simulink model "base_1fm"  (R2016b)
settings: Solver=VariableStepAuto  StartTime=0.0  StopTime=10.0  RelTol=1e-3
values from neighbouring files (symbols this model uses):
  Lb = 0.07    [base_1fm_parameters.m]
  Lf = 0.238    [base_1fm_parameters.m]
  Lu = 0.153    [base_1fm_parameters.m]
  sampleTime = 0.001    [base_1fm_parameters.m]
undefined symbols (not defined in the file or in its folder): DiscIntNeverNeededParam, RobotStruct
undefined symbols (not defined in the file): RobotStruct_FM1
libraries: simulink x27, VariousBlocksLibrary x4, FMLibrary_v2 x2, UsefulBlocksLibrary x2, simulink_extras x2, FM_Library x1
(part 1 of 3)
settings Model: Creator=niekbeckers  LastModifiedBy=niekbeckers

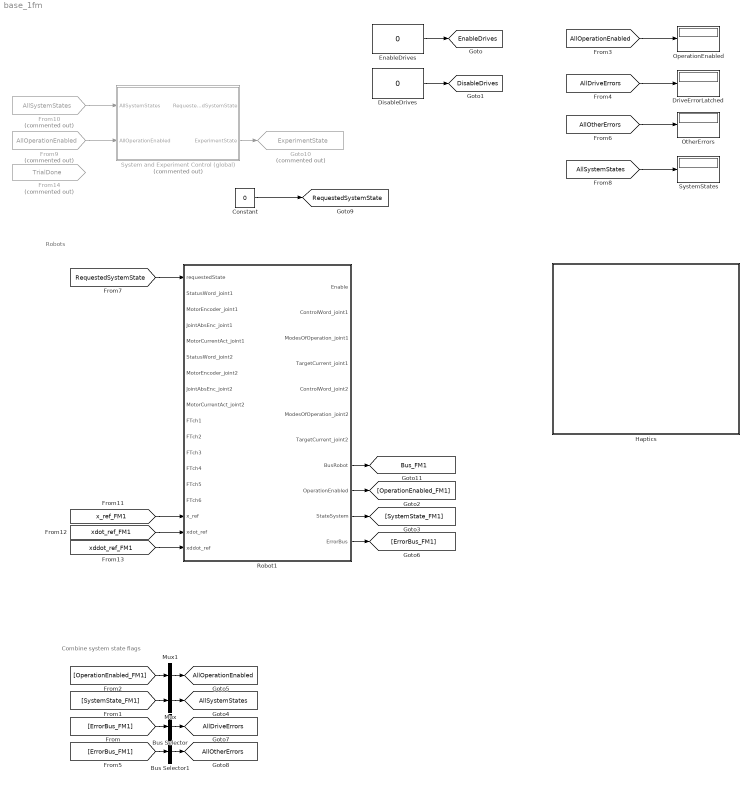
== system base_1fm ==
  note: Combine system state flags
  note: Robots
  Bus Selector : BusSelector  OutputSignals=DriveErrorLatched  OutputAsBus=on
  Bus Selector1 : BusSelector  OutputSignals=WorkspaceErrorLatched,ForceSensorLatched  OutputAsBus=on
  Constant : Constant  Value=0
  DisableDrives : Constant  Value=0
      settings: OpenFcn=set_param(gcb,'Value','1');tname = ['toggletimer_' gcb];delete(timerfind('name',tname));t = timer('timerfcn', ['set_param(''',gcb,''',''Value'',''0'')'],'executionmode','singleshot','startdelay',1,'name',tname);start(t);
      mask Display: fprintf('PushToTrigger\n%s',get_param(gcb,'value'))
  DriveErrorLatched : Display
  EnableDrives : Constant  Value=0
      settings: OpenFcn=set_param(gcb,'Value','1');tname = ['toggletimer_' gcb];delete(timerfind('name',tname));t = timer('timerfcn', ['set_param(''',gcb,''',''Value'',''0'')'],'executionmode','singleshot','startdelay',1,'name',tname);start(t);
      mask Display: fprintf('PushToTrigger\n%s',get_param(gcb,'value'))
  From10 : From  Commented=on  GotoTag=AllSystemStates
  From14 : From  Commented=on  GotoTag=TrialDone
  From9 : From  Commented=on  GotoTag=AllOperationEnabled
  Goto10 : Goto  Commented=on  GotoTag=ExperimentState  TagVisibility=global
  Haptics : Subsystem
  Mux : Mux  Inputs=1
  Mux1 : Mux  Inputs=1
  OperationEnabled : Display
  OtherErrors : Display
  Robot1 : Subsystem  mask{RobotStruct=RobotStruct_FM1}
      mask prompts: RobotStruct "Robot struct (data)"
  System and Experiment Control (global) : Subsystem  Commented=on
  SystemStates : Display
  tag scope: AllDriveErrors=global, AllOperationEnabled=global, AllOtherErrors=global, AllSystemStates=global, Bus_FM1=global, DisableDrives=global, EnableDrives=global, RequestedSystemState=global
  wires:
  DisableDrives/1 -> [DisableDrives]
  EnableDrives/1 -> [EnableDrives]
  Robot1/9(OperationEnabled) -> [OperationEnabled_FM1]
  [AllOperationEnabled] -> OperationEnabled/1
  Robot1/10(StateSystem) -> [SystemState_FM1]
  [SystemState_FM1] -> Mux/1
  Mux/1 -> [AllSystemStates]
  Mux1/1 -> [AllOperationEnabled]
  [OperationEnabled_FM1] -> Mux1/1
  Robot1/11(ErrorBus) -> [ErrorBus_FM1]
  [ErrorBus_FM1] -> Bus Selector/1
  Bus Selector/1 -> [AllDriveErrors]
  [AllDriveErrors] -> DriveErrorLatched/1
  [ErrorBus_FM1] -> Bus Selector1/1
  Bus Selector1/1 -> [AllOtherErrors]
  [AllOtherErrors] -> OtherErrors/1
  [RequestedSystemState] -> Robot1/1(requestedState)
  [AllSystemStates] -> SystemStates/1
  System and Experiment Control (global)/2(ExperimentState) -> Goto10/1
  From10/1 -> System and Experiment Control (global)/1(AllSystemStates)
  From9/1 -> System and Experiment Control (global)/2(AllOperationEnabled)
  [x_ref_FM1] -> Robot1/16(x_ref)
  [xdot_ref_FM1] -> Robot1/17(xdot_ref)
  [xddot_ref_FM1] -> Robot1/18(xddot_ref)
  Constant/1 -> [RequestedSystemState]
  Robot1/8(BusRobot) -> [Bus_FM1]

== system base_1fm/Haptics ==
  note: Only run trajectory if all systems are in state 4 (run)
  Add : Sum
  "Check state " : simulink/Logic and Bit Operations/Compare To Constant  relop===  const=4  OutDataTypeStr=boolean
  Constant : Constant  Value=RobotStruct.HomeLocationOpSpace
  From9 : From  Commented=on  GotoTag=ExperimentState
  Goto1 : Goto  Commented=on  GotoTag=TrialDone  TagVisibility=global
  Hypotrochoid trajectory for AFFC : Subsystem
  Logical Operator : Logic  Inputs=1  AllPortsSameDT=off  OutDataTypeStr=boolean
  Terminator : Terminator
  Terminator1 : Terminator  Commented=on
  tag scope: x_ref_FM1=global, xddot_ref_FM1=global, xdot_ref_FM1=global
  wires:
  [Bus_FM1] -> Terminator/1
  Constant/1 -> Add/1
  Hypotrochoid trajectory for AFFC/1(dx_ref) -> Add/2
  Add/1 -> [x_ref_FM1]
  Hypotrochoid trajectory for AFFC/2(dxdot_ref) -> [xdot_ref_FM1]
  Hypotrochoid trajectory for AFFC/3(dxddot_ref) -> [xddot_ref_FM1]
  [AllSystemStates] -> "Check state "/1
  "Check state "/1 -> Logical Operator/1
  Logical Operator/1 -> Hypotrochoid trajectory for AFFC/Enable
  From9/1 -> Terminator1/1

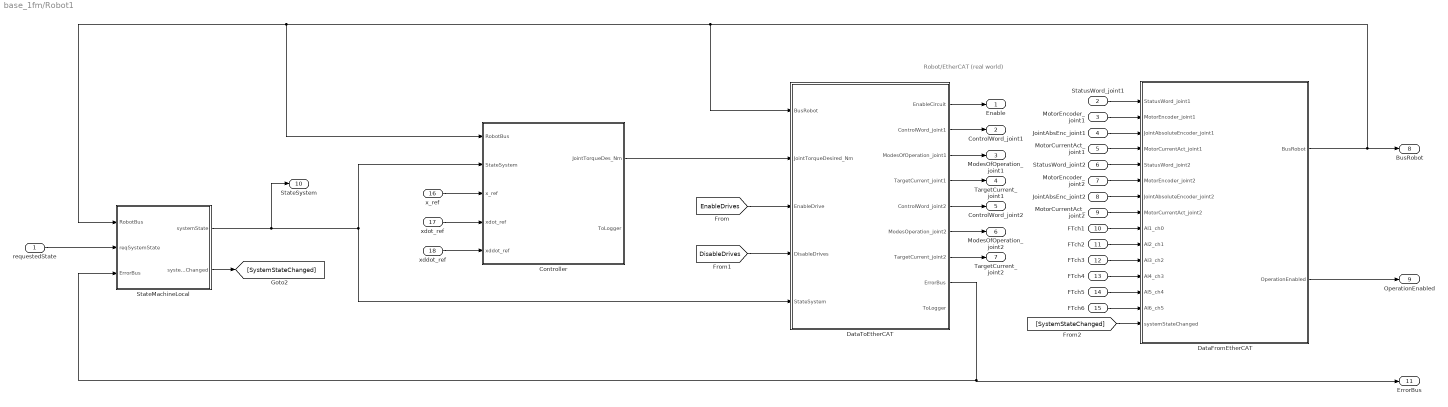
== system base_1fm/Robot1 ==
  note: Robot/EtherCAT (real world)
  requestedState : Inport
  StatusWord_joint1 : Inport  Port=2
  MotorEncoder_joint1 : Inport  Port=3
  JointAbsEnc_joint1 : Inport  Port=4
  MotorCurrentAct_joint1 : Inport  Port=5
  StatusWord_joint2 : Inport  Port=6
  MotorEncoder_joint2 : Inport  Port=7
  JointAbsEnc_joint2 : Inport  Port=8
  MotorCurrentAct_joint2 : Inport  Port=9
  FTch1 : Inport  Port=10
  FTch2 : Inport  Port=11
  FTch3 : Inport  Port=12
  FTch4 : Inport  Port=13
  FTch5 : Inport  Port=14
  FTch6 : Inport  Port=15
  x_ref : Inport  Port=16
  xdot_ref : Inport  Port=17
  xddot_ref : Inport  Port=18
  Controller : Subsystem  AncestorBlock=FMLibrary_v2/Controller
  DataFromEtherCAT : Subsystem  AncestorBlock=FMLibrary_v2/DataFromEtherCAT_FM
  DataToEtherCAT : Subsystem  AncestorBlock=FMLibrary_v2/DataToEtherCAT_FM
  StateMachineLocal : Subsystem  AncestorBlock=FMLibrary_v2/StateMachineLocal
  Enable : Outport
  ControlWord_joint1 : Outport  Port=2
  ModesOfOperation_joint1 : Outport  Port=3
  TargetCurrent_joint1 : Outport  Port=4
  ControlWord_joint2 : Outport  Port=5
  ModesOfOperation_joint2 : Outport  Port=6
  TargetCurrent_joint2 : Outport  Port=7
  BusRobot : Outport  Port=8
  OperationEnabled : Outport  Port=9
  StateSystem : Outport  Port=10
  ErrorBus : Outport  Port=11
  wires:
  DataFromEtherCAT/2(OperationEnabled) -> OperationEnabled/1
  FTch3/1 -> DataFromEtherCAT/11(AI3_ch2)
  FTch4/1 -> DataFromEtherCAT/12(AI4_ch3)
  FTch6/1 -> DataFromEtherCAT/14(AI6_ch5)
  StatusWord_joint2/1 -> DataFromEtherCAT/5(StatusWord_joint2)
  StatusWord_joint1/1 -> DataFromEtherCAT/1(StatusWord_joint1)
  DataToEtherCAT/6(ModesOperation_joint2) -> ModesOfOperation_joint2/1
  DataToEtherCAT/5(ControlWord_joint2) -> ControlWord_joint2/1
  MotorEncoder_joint1/1 -> DataFromEtherCAT/2(MotorEncoder_joint1)
  JointAbsEnc_joint2/1 -> DataFromEtherCAT/7("JointAbsoluteEncoder_joint2 ")
  FTch5/1 -> DataFromEtherCAT/13(AI5_ch4)
  DataToEtherCAT/4(TargetCurrent_joint1) -> TargetCurrent_joint1/1
  MotorCurrentAct_joint2/1 -> DataFromEtherCAT/8(MotorCurrentAct_joint2)
  [EnableDrives] -> DataToEtherCAT/3(EnableDrive)
  [DisableDrives] -> DataToEtherCAT/4(DisableDrives)
  Controller/1(JointTorqueDes_Nm) -> DataToEtherCAT/2(JointTorqueDesired_Nm)
  requestedState/1 -> StateMachineLocal/2(reqSystemState)
  DataFromEtherCAT/1(BusRobot) -> BusRobot/1, DataToEtherCAT/1(BusRobot), Controller/1(RobotBus), StateMachineLocal/1(RobotBus)
  DataToEtherCAT/8(ErrorBus) -> ErrorBus/1, StateMachineLocal/3(ErrorBus)
  [SystemStateChanged] -> DataFromEtherCAT/15(systemStateChanged)
  StateMachineLocal/2(systemStateChanged) -> [SystemStateChanged]
  DataToEtherCAT/2(ControlWord_joint1) -> ControlWord_joint1/1
  StateMachineLocal/1(systemState) -> StateSystem/1, DataToEtherCAT/5(StateSystem), Controller/2(StateSystem)
  FTch1/1 -> DataFromEtherCAT/9(AI1_ch0)
  DataToEtherCAT/1(EnableCircuit) -> Enable/1
  DataToEtherCAT/3(ModesOfOperation_joint1) -> ModesOfOperation_joint1/1
  JointAbsEnc_joint1/1 -> DataFromEtherCAT/3(JointAbsoluteEncoder_joint1)
  MotorEncoder_joint2/1 -> DataFromEtherCAT/6(MotorEncoder_joint2)
  MotorCurrentAct_joint1/1 -> DataFromEtherCAT/4(MotorCurrentAct_joint1)
  FTch2/1 -> DataFromEtherCAT/10(AI2_ch1)
  DataToEtherCAT/7(TargetCurrent_joint2) -> TargetCurrent_joint2/1
  x_ref/1 -> Controller/3(x_ref)
  xdot_ref/1 -> Controller/4(xdot_ref)
  xddot_ref/1 -> Controller/5(xddot_ref)

== system base_1fm/System and Experiment Control (global) ==
  note: Hier ergens experiment protocol inlezen
  AllSystemStates : Inport
  AllOperationEnabled : Inport  Port=2
  GlobalStateMachine : FMLibrary_v2/StateMachineLocal/SystemLocalStateMachine
  RequestedSystemState : Outport
  ExperimentState : Outport  Port=2
  wires:
  GlobalStateMachine/1 -> RequestedSystemState/1

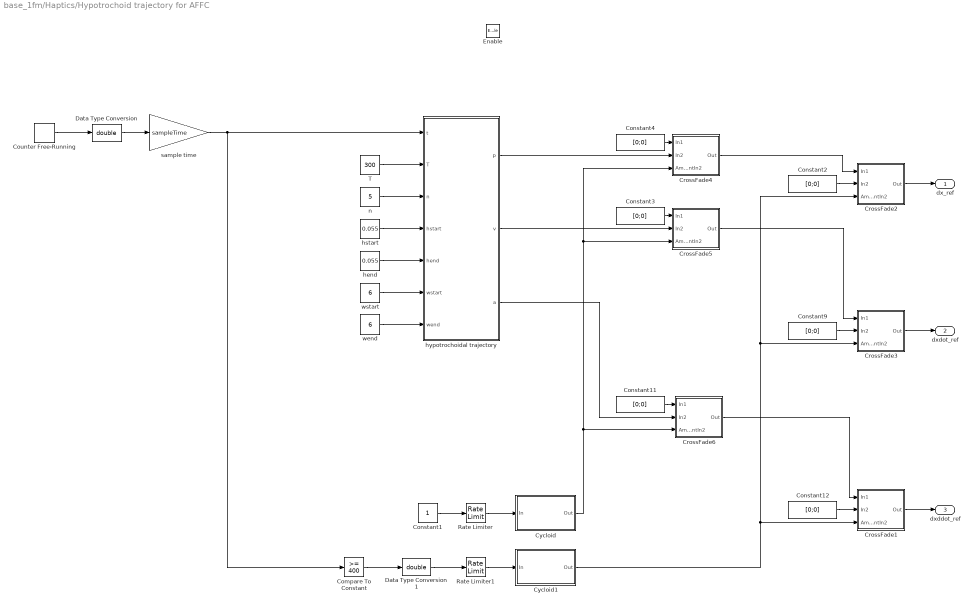
== system base_1fm/Haptics/Hypotrochoid trajectory for AFFC ==
  Enable : EnablePort  StatesWhenEnabling=reset
  Compare To Constant : simulink/Logic and Bit Operations/Compare To Constant  relop=>=  const=400  OutDataTypeStr=boolean
  Constant1 : Constant
  Constant{2..4,9,11..12} (6 alike) : Constant  Value=[0;0]
  Counter Free-Running : simulink/Sources/Counter Free-Running  NumBits=32  tsamp=-1
  CrossFade1 : Subsystem  AncestorBlock=VariousBlocksLibrary/Various/CrossFade
  CrossFade2 : Subsystem  AncestorBlock=VariousBlocksLibrary/Various/CrossFade
  CrossFade3 : Subsystem  AncestorBlock=VariousBlocksLibrary/Various/CrossFade
  CrossFade4 : Subsystem  AncestorBlock=VariousBlocksLibrary/Various/CrossFade
  CrossFade5 : Subsystem  AncestorBlock=VariousBlocksLibrary/Various/CrossFade
  CrossFade6 : Subsystem  AncestorBlock=VariousBlocksLibrary/Various/CrossFade
  Cycloid : Subsystem  AncestorBlock=VariousBlocksLibrary/Various/Cycloid
  Cycloid1 : Subsystem  AncestorBlock=VariousBlocksLibrary/Various/Cycloid
  Data Type Conversion : DataTypeConversion  OutDataTypeStr=double
  Data Type Conversion1 : DataTypeConversion  OutDataTypeStr=double
  Rate Limiter : RateLimiter  RisingSlewLimit=0.25  FallingSlewLimit=-0.15  SampleTimeMode=inherited
  Rate Limiter1 : RateLimiter  RisingSlewLimit=0.2  FallingSlewLimit=-0.2  SampleTimeMode=inherited
  T : Constant  Value=300
  hend : Constant  Value=0.055
  hstart : Constant  Value=0.055
  hypotrochoidal trajectory : MATLAB Function  TreatAsAtomicUnit=on
  n : Constant  Value=5
  sample time : Gain  Gain=sampleTime
  wend : Constant  Value=6
  wstart : Constant  Value=6
  dx_ref : Outport
  dxdot_ref : Outport  Port=2
  dxddot_ref : Outport  Port=3
  wires:
  Data Type Conversion1/1 -> Rate Limiter1/1
  hypotrochoidal trajectory/1(p) -> CrossFade4/2(In2)
  CrossFade1/1(Out) -> dxddot_ref/1
  Constant11/1 -> CrossFade6/1(In1)
  Constant12/1 -> CrossFade1/2(In2)
  CrossFade6/1(Out) -> CrossFade1/1(In1)
  Constant9/1 -> CrossFade3/2(In2)
  CrossFade5/1(Out) -> CrossFade3/1(In1)
  CrossFade3/1(Out) -> dxdot_ref/1
  Cycloid1/1(Out) -> CrossFade1/3(AmountIn2), CrossFade2/3(AmountIn2), CrossFade3/3(AmountIn2)
  Rate Limiter1/1 -> Cycloid1/1(In)
  Compare To Constant/1 -> Data Type Conversion1/1
  CrossFade4/1(Out) -> CrossFade2/1(In1)
  CrossFade2/1(Out) -> dx_ref/1
  Rate Limiter/1 -> Cycloid/1(In)
  Constant1/1 -> Rate Limiter/1
  Cycloid/1(Out) -> CrossFade6/3(AmountIn2), CrossFade5/3(AmountIn2), CrossFade4/3(AmountIn2)
  hypotrochoidal trajectory/2(v) -> CrossFade5/2(In2)
  hypotrochoidal trajectory/3(a) -> CrossFade6/2(In2)
  sample time/1 -> Compare To Constant/1, hypotrochoidal trajectory/1(t)
  Constant2/1 -> CrossFade2/2(In2)
  Data Type Conversion/1 -> sample time/1
  wstart/1 -> hypotrochoidal trajectory/6(wstart)
  wend/1 -> hypotrochoidal trajectory/7(wend)
  hstart/1 -> hypotrochoidal trajectory/4(hstart)
  hend/1 -> hypotrochoidal trajectory/5(hend)
  n/1 -> hypotrochoidal trajectory/3(n)
  T/1 -> hypotrochoidal trajectory/2(T)
  Counter Free-Running/1 -> Data Type Conversion/1
  Constant3/1 -> CrossFade5/1(In1)
  Constant4/1 -> CrossFade4/1(In1)

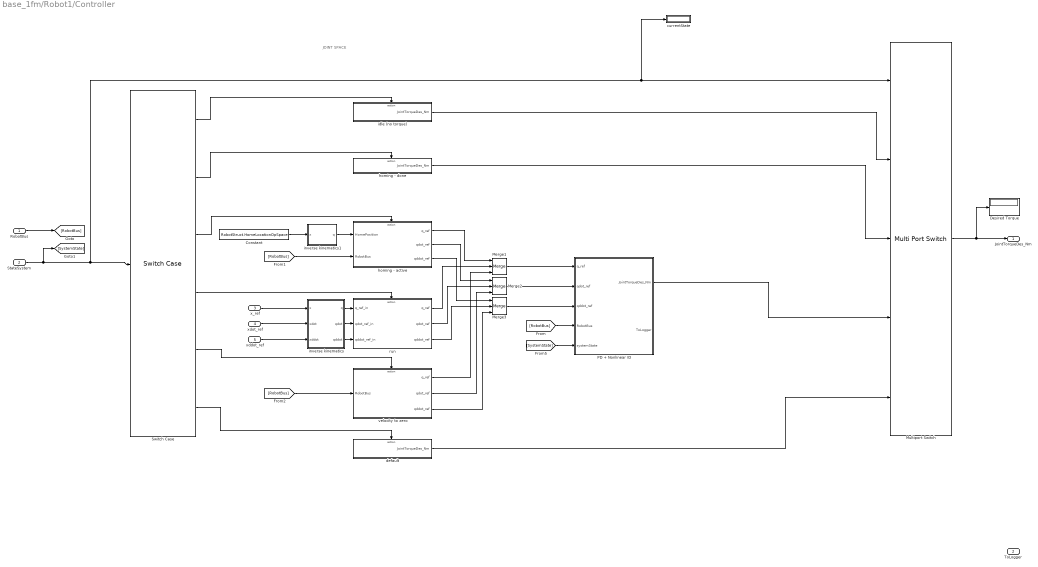
== system base_1fm/Robot1/Controller ==
  note: JOINT SPACE
  RobotBus : Inport
  StateSystem : Inport  Port=2
  x_ref : Inport  Port=3
  xdot_ref : Inport  Port=4
  xddot_ref : Inport  Port=5
  Constant : Constant  Value=RobotStruct.HomeLocationOpSpace
  Desired Torque : Display
  Merge1 : Merge  Inputs=3
  Merge2 : Merge  Inputs=3
  Merge3 : Merge  Inputs=3
  Multiport Switch : MultiPortSwitch  DataPortOrder=Specify indices  Inputs=4  DataPortIndices={[0,1,2,201,299,301],[399],[302,4]}  DataPortForDefault=Additional data port
  PD + Nonlinear ID : Subsystem
  Switch Case : SwitchCase  CaseConditions={[0,1,2,201,299,301],[399],[302],[4],[499]}
  currentState : Display
  default : Subsystem  TreatAsAtomicUnit=on
  homing - active : Subsystem
  homing - done : Subsystem  TreatAsAtomicUnit=on
  idle (no torque) : Subsystem  TreatAsAtomicUnit=on
  inverse kinematics : MATLAB Function  TreatAsAtomicUnit=on
  inverse kinematics1 : MATLAB Function  TreatAsAtomicUnit=on
  run : Subsystem
  velocity to zero : Subsystem
  JointTorqueDes_Nm : Outport
  ToLogger : Outport  Port=2
  wires:
  homing - active/3(qddot_ref) -> Merge3/1
  homing - active/2(qdot_ref) -> Merge2/1
  run/3(qddot_ref) -> Merge3/2
  run/2(qdot_ref) -> Merge2/2
  StateSystem/1 -> [SystemState], Switch Case/1, currentState/1, Multiport Switch/1
  run/1(q_ref) -> Merge1/2
  homing - active/1(q_ref) -> Merge1/1
  Switch Case/4 -> run/Action
  Multiport Switch/1 -> JointTorqueDes_Nm/1, Desired Torque/1
  Switch Case/6 -> default/Action
  default/1(JointTorqueDes_Nm) -> Multiport Switch/5
  Switch Case/1 -> idle (no torque)/Action
  Switch Case/3 -> homing - active/Action
  Switch Case/2 -> homing - done/Action
  idle (no torque)/1(JointTorqueDes_Nm) -> Multiport Switch/2
  homing - done/1(JointTorqueDes_Nm) -> Multiport Switch/3
  Merge1/1 -> PD + Nonlinear ID/1(q_ref)
  Merge2/1 -> PD + Nonlinear ID/2(qdot_ref)
  Merge3/1 -> PD + Nonlinear ID/3(qddot_ref)
  PD + Nonlinear ID/1(JointTorqueDes_Nm) -> Multiport Switch/4
  RobotBus/1 -> [RobotBus]
  [RobotBus] -> PD + Nonlinear ID/4(RobotBus)
  [RobotBus] -> homing - active/2(RobotBus)
  Constant/1 -> inverse kinematics1/1(x)
  inverse kinematics/1(q) -> run/1(q_ref_in)
  inverse kinematics/2(qdot) -> run/2(qdot_ref_in)
  inverse kinematics/3(qddot) -> run/3(qddot_ref_in)
  inverse kinematics1/1(q) -> homing - active/1(HomePosition)
  [SystemState] -> PD + Nonlinear ID/5(systemState)
  x_ref/1 -> inverse kinematics/1(x)
  xddot_ref/1 -> inverse kinematics/3(xddot)
  xdot_ref/1 -> inverse kinematics/2(xdot)
  velocity to zero/1(q_ref) -> Merge1/3
  velocity to zero/2(qdot_ref) -> Merge2/3
  velocity to zero/3(qddot_ref) -> Merge3/3
  Switch Case/5 -> velocity to zero/Action
  [RobotBus] -> velocity to zero/1(RobotBus)

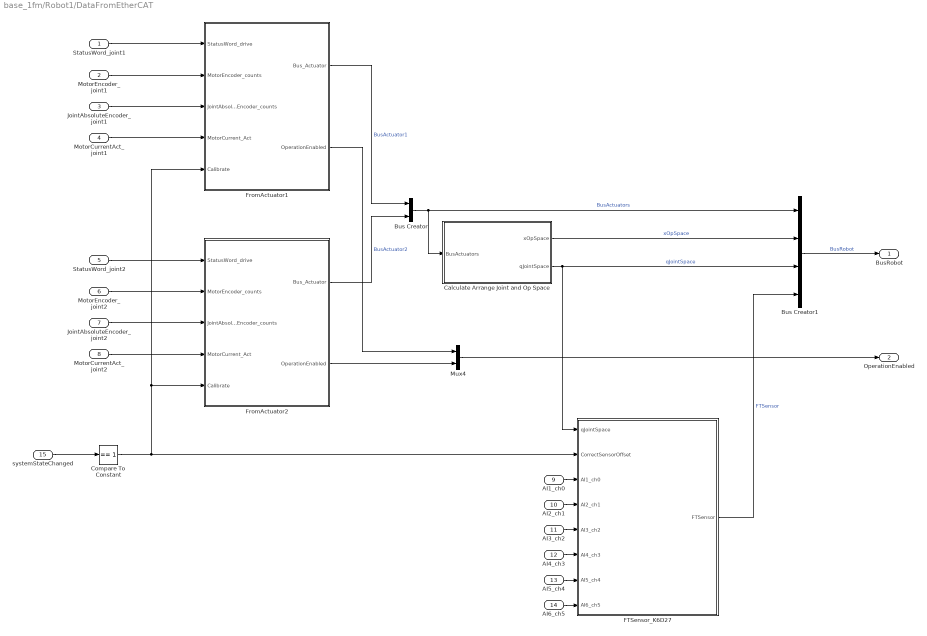
== system base_1fm/Robot1/DataFromEtherCAT ==
  StatusWord_joint1 : Inport
  MotorEncoder_joint1 : Inport  Port=2
  JointAbsoluteEncoder_joint1 : Inport  Port=3
  MotorCurrentAct_joint1 : Inport  Port=4
  StatusWord_joint2 : Inport  Port=5
  MotorEncoder_joint2 : Inport  Port=6
  "JointAbsoluteEncoder_joint2 " : Inport  Port=7
  MotorCurrentAct_joint2 : Inport  Port=8
  AI1_ch0 : Inport  Port=9  OutDataTypeStr=int16
  AI2_ch1 : Inport  Port=10  OutDataTypeStr=int16
  AI3_ch2 : Inport  Port=11  OutDataTypeStr=int16
  AI4_ch3 : Inport  Port=12  OutDataTypeStr=int16
  AI5_ch4 : Inport  Port=13  OutDataTypeStr=int16
  AI6_ch5 : Inport  Port=14  OutDataTypeStr=int16
  systemStateChanged : Inport  Port=15
  Bus Creator : BusCreator  Inputs=2
  Bus Creator1 : BusCreator  Inputs=4
  Calculate Arrange Joint and Op Space : Subsystem
  Compare To Constant : simulink/Logic and Bit Operations/Compare To Constant  relop===  const=1  OutDataTypeStr=boolean
  FTSensor_K6D27 : Subsystem  mask{FTSensorStruct=RobotStruct.FTSensor}
      mask prompts: FTSensorStruct "Struct for force torque sensor"
  FromActuator1 : Subsystem  AncestorBlock=FMLibrary_v2/FromActuator1  mask{ActuatorStruct=RobotStruct.Actuator1}
      mask prompts: ActuatorStruct "Actuator Struct"
  FromActuator2 : Subsystem  AncestorBlock=FMLibrary_v2/FromActuator1  mask{ActuatorStruct=RobotStruct.Actuator2}
      mask prompts: ActuatorStruct "Actuator Struct"
  Mux4 : Mux  Inputs=2
  BusRobot : Outport
  OperationEnabled : Outport  Port=2
  wires:
  Compare To Constant/1 -> FTSensor_K6D27/2(CorrectSensorOffset), FromActuator1/5(Calibrate), FromActuator2/5(Calibrate)
  FTSensor_K6D27/1(FTSensor) -> Bus Creator1/4  "FTSensor"
  AI6_ch5/1 -> FTSensor_K6D27/8(AI6_ch5)
  AI5_ch4/1 -> FTSensor_K6D27/7(AI5_ch4)
  AI4_ch3/1 -> FTSensor_K6D27/6(AI4_ch3)
  AI3_ch2/1 -> FTSensor_K6D27/5(AI3_ch2)
  AI2_ch1/1 -> FTSensor_K6D27/4(AI2_ch1)
  AI1_ch0/1 -> FTSensor_K6D27/3(AI1_ch0)
  systemStateChanged/1 -> Compare To Constant/1
  Calculate Arrange Joint and Op Space/2(qJointSpace) -> Bus Creator1/3, FTSensor_K6D27/1(qJointSpace)  "qJointSpace"
  Calculate Arrange Joint and Op Space/1(xOpSpace) -> Bus Creator1/2  "xOpSpace"
  Bus Creator1/1 -> BusRobot/1  "BusRobot"
  Bus Creator/1 -> Bus Creator1/1, Calculate Arrange Joint and Op Space/1(BusActuators)  "BusActuators"
  MotorCurrentAct_joint2/1 -> FromActuator2/4(MotorCurrent_Act)
  "JointAbsoluteEncoder_joint2 "/1 -> FromActuator2/3(JointAbsoluteEncoder_counts)
  StatusWord_joint2/1 -> FromActuator2/1(StatusWord_drive)
  MotorEncoder_joint2/1 -> FromActuator2/2(MotorEncoder_counts)
  MotorCurrentAct_joint1/1 -> FromActuator1/4(MotorCurrent_Act)
  JointAbsoluteEncoder_joint1/1 -> FromActuator1/3(JointAbsoluteEncoder_counts)
  StatusWord_joint1/1 -> FromActuator1/1(StatusWord_drive)
  MotorEncoder_joint1/1 -> FromActuator1/2(MotorEncoder_counts)
  FromActuator2/2(OperationEnabled) -> Mux4/2
  Mux4/1 -> OperationEnabled/1
  FromActuator1/2(OperationEnabled) -> Mux4/1
  FromActuator2/1(Bus_Actuator) -> Bus Creator/2  "BusActuator2"
  FromActuator1/1(Bus_Actuator) -> Bus Creator/1  "BusActuator1"

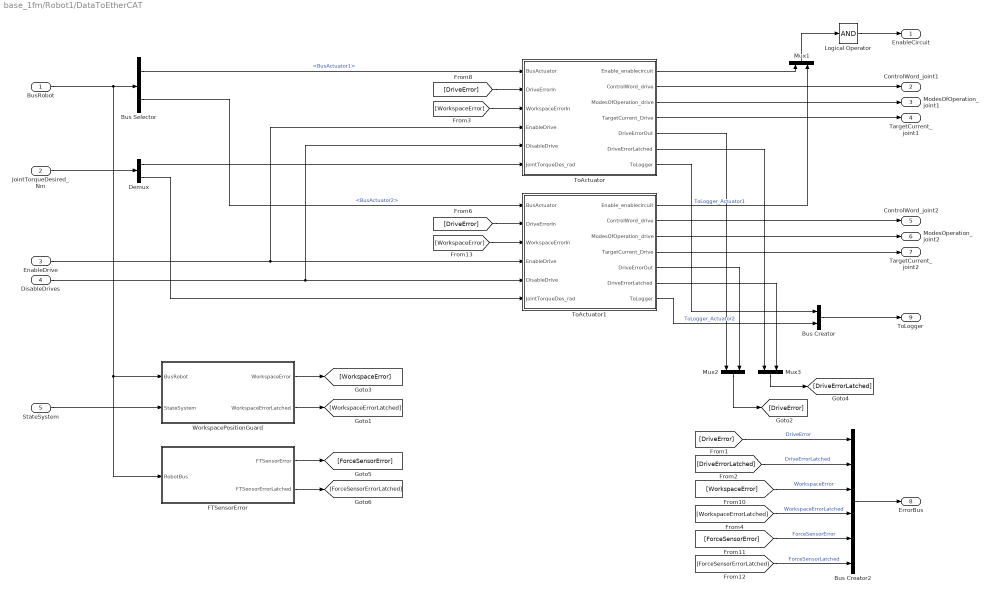
== system base_1fm/Robot1/DataToEtherCAT ==
  BusRobot : Inport
  JointTorqueDesired_Nm : Inport  Port=2
  EnableDrive : Inport  Port=3
  DisableDrives : Inport  Port=4
  StateSystem : Inport  Port=5
  Bus Creator : BusCreator  Inputs=2
  Bus Creator2 : BusCreator  Inputs=6
  Bus Selector : BusSelector  OutputSignals=BusActuators.BusActuator1,BusActuators.BusActuator2
  Demux : Demux  Outputs=2
  FTSensorError : Subsystem
  Logical Operator : Logic  Inputs=1  AllPortsSameDT=off  OutDataTypeStr=boolean
  Mux1 : Mux  Inputs=2
  Mux2 : Mux  Inputs=2
  Mux3 : Mux  Inputs=2
  ToActuator : Subsystem  AncestorBlock=FMLibrary_v2/ToActuator  mask{ActuatorStruct=RobotStruct.Actuator1}
      mask prompts: ActuatorStruct "Actuator Struct"
  ToActuator1 : Subsystem  AncestorBlock=FMLibrary_v2/ToActuator  mask{ActuatorStruct=RobotStruct.Actuator2}
      mask prompts: ActuatorStruct "Actuator Struct"
  WorkspacePositionGuard : Subsystem
  EnableCircuit : Outport
  ControlWord_joint1 : Outport  Port=2
  ModesOfOperation_joint1 : Outport  Port=3
  TargetCurrent_joint1 : Outport  Port=4
  ControlWord_joint2 : Outport  Port=5
  ModesOperation_joint2 : Outport  Port=6
  TargetCurrent_joint2 : Outport  Port=7
  ErrorBus : Outport  Port=8
  ToLogger : Outport  Port=9
  wires:
  [ForceSensorErrorLatched] -> Bus Creator2/6  "ForceSensorLatched"
  [ForceSensorError] -> Bus Creator2/5  "ForceSensorError"
  FTSensorError/2(FTSensorErrorLatched) -> [ForceSensorErrorLatched]
  FTSensorError/1(FTSensorError) -> [ForceSensorError]
  StateSystem/1 -> WorkspacePositionGuard/2(StateSystem)
  [WorkspaceErrorLatched] -> Bus Creator2/4  "WorkspaceErrorLatched"
  [WorkspaceError] -> Bus Creator2/3  "WorkspaceError"
  [DriveErrorLatched] -> Bus Creator2/2  "DriveErrorLatched"
  [DriveError] -> Bus Creator2/1  "DriveError"
  Bus Creator2/1 -> ErrorBus/1
  Mux3/1 -> [DriveErrorLatched]
  [WorkspaceError] -> ToActuator1/3(WorkspaceErrorIn)
  [DriveError] -> ToActuator1/2(DriveErrorIn)
  EnableDrive/1 -> ToActuator1/4(EnableDrive), ToActuator/4(EnableDrive)
  DisableDrives/1 -> ToActuator1/5(DisableDrive), ToActuator/5(DisableDrive)
  [WorkspaceError] -> ToActuator/3(WorkspaceErrorIn)
  WorkspacePositionGuard/1(WorkspaceError) -> [WorkspaceError]
  WorkspacePositionGuard/2(WorkspaceErrorLatched) -> [WorkspaceErrorLatched]
  Bus Selector/1 -> ToActuator/1(BusActuator)  "<BusActuator1>"
  Bus Selector/2 -> ToActuator1/1(BusActuator)  "<BusActuator2>"
  BusRobot/1 -> Bus Selector/1, WorkspacePositionGuard/1(BusRobot), FTSensorError/1(RobotBus)
  Demux/1 -> ToActuator/6(JointTorqueDes_rad)
  JointTorqueDesired_Nm/1 -> Demux/1
  Demux/2 -> ToActuator1/6(JointTorqueDes_rad)
  Logical Operator/1 -> EnableCircuit/1
  ToActuator1/3(ModesOfOperation_drive) -> ModesOperation_joint2/1
  ToActuator1/4(TargetCurrent_Drive) -> TargetCurrent_joint2/1
  ToActuator/4(TargetCurrent_Drive) -> TargetCurrent_joint1/1
  ToActuator1/2(ControlWord_drive) -> ControlWord_joint2/1
  ToActuator/3(ModesOfOperation_drive) -> ModesOfOperation_joint1/1
  ToActuator/2(ControlWord_drive) -> ControlWord_joint1/1
  ToActuator1/1(Enable_enablecircuit) -> Mux1/2
  ToActuator/1(Enable_enablecircuit) -> Mux1/1
  Mux1/1 -> Logical Operator/1
  [DriveError] -> ToActuator/2(DriveErrorIn)
  ToActuator1/6(DriveErrorLatched) -> Mux3/2
  ToActuator/6(DriveErrorLatched) -> Mux3/1
  Mux2/1 -> [DriveError]
  ToActuator1/5(DriveErrorOut) -> Mux2/2
  ToActuator/5(DriveErrorOut) -> Mux2/1
  ToActuator/7(ToLogger) -> Bus Creator/1  "ToLogger_Actuator1"
  ToActuator1/7(ToLogger) -> Bus Creator/2  "ToLogger_Actuator2"
  Bus Creator/1 -> ToLogger/1

== system base_1fm/Robot1/StateMachineLocal ==
  note: Encode system state change - powers of 2 indicate which state change occurs.
  RobotBus : Inport
  reqSystemState : Inport  Port=2
  ErrorBus : Inport  Port=3
  Bus Selector : BusSelector  OutputSignals=xOpSpace.x,xOpSpace.xdot
  Constant : Constant  Value=RobotStruct.HomeLocationSize
  Constant1 : Constant  Value=RobotStruct.HomeLocationOpSpace
  Detect Change1 : simulink/Logic and Bit Operations/Detect Change  vinit=0  InputProcessing=Inherited  OutDataTypeStr=boolean
  Encode system state change : MATLAB Function  TreatAsAtomicUnit=on
  SystemLocalStateMachine : Stateflow chart  TreatAsAtomicUnit=on
  systemState : Outport
  systemStateChanged : Outport  Port=2
  wires:
  Bus Selector/2 -> SystemLocalStateMachine/4(xdot)  "<xdot>"
  Bus Selector/1 -> SystemLocalStateMachine/3(x)  "<x>"
  RobotBus/1 -> Bus Selector/1
  Constant1/1 -> SystemLocalStateMachine/5(HomePosition)
  Constant/1 -> SystemLocalStateMachine/6(homeLocationSize)
  Encode system state change/1(systemStateChanged) -> systemStateChanged/1
  Detect Change1/1 -> Encode system state change/1(stateChanged)
  ErrorBus/1 -> SystemLocalStateMachine/2(error)
  SystemLocalStateMachine/1(currentSystemState) -> Encode system state change/2(state), Detect Change1/1, systemState/1
  reqSystemState/1 -> SystemLocalStateMachine/1(reqSystemState)

== system base_1fm/Haptics/Hypotrochoid trajectory for AFFC/CrossFade1 ==
  In1 : Inport
  In2 : Inport  Port=2
  AmountIn2 : Inport  Port=3
  Add : Sum  Inputs=+-
  Add1 : Sum
  One : Constant
  Product : Product  RndMeth=Zero
  Product1 : Product  RndMeth=Zero
  Saturation : Saturate  UpperLimit=1  LowerLimit=0
  Out : Outport
  wires:
  In1/1 -> Product1/1
  AmountIn2/1 -> Saturation/1
  One/1 -> Add/1
  Saturation/1 -> Product/2, Add/2
  Add/1 -> Product1/2
  Product/1 -> Add1/2
  Product1/1 -> Add1/1
  In2/1 -> Product/1
  Add1/1 -> Out/1

== system base_1fm/Haptics/Hypotrochoid trajectory for AFFC/CrossFade2 ==
  In1 : Inport
  In2 : Inport  Port=2
  AmountIn2 : Inport  Port=3
  Add : Sum  Inputs=+-
  Add1 : Sum
  One : Constant
  Product : Product  RndMeth=Zero
  Product1 : Product  RndMeth=Zero
  Saturation : Saturate  UpperLimit=1  LowerLimit=0
  Out : Outport
  wires:
  In1/1 -> Product1/1
  AmountIn2/1 -> Saturation/1
  One/1 -> Add/1
  Saturation/1 -> Product/2, Add/2
  Add/1 -> Product1/2
  Product/1 -> Add1/2
  Product1/1 -> Add1/1
  In2/1 -> Product/1
  Add1/1 -> Out/1

== system base_1fm/Haptics/Hypotrochoid trajectory for AFFC/CrossFade3 ==
  In1 : Inport
  In2 : Inport  Port=2
  AmountIn2 : Inport  Port=3
  Add : Sum  Inputs=+-
  Add1 : Sum
  One : Constant
  Product : Product  RndMeth=Zero
  Product1 : Product  RndMeth=Zero
  Saturation : Saturate  UpperLimit=1  LowerLimit=0
  Out : Outport
  wires:
  In1/1 -> Product1/1
  AmountIn2/1 -> Saturation/1
  One/1 -> Add/1
  Saturation/1 -> Product/2, Add/2
  Add/1 -> Product1/2
  Product/1 -> Add1/2
  Product1/1 -> Add1/1
  In2/1 -> Product/1
  Add1/1 -> Out/1

== system base_1fm/Haptics/Hypotrochoid trajectory for AFFC/CrossFade4 ==
  In1 : Inport
  In2 : Inport  Port=2
  AmountIn2 : Inport  Port=3
  Add : Sum  Inputs=+-
  Add1 : Sum
  One : Constant
  Product : Product  RndMeth=Zero
  Product1 : Product  RndMeth=Zero
  Saturation : Saturate  UpperLimit=1  LowerLimit=0
  Out : Outport
  wires:
  In1/1 -> Product1/1
  AmountIn2/1 -> Saturation/1
  One/1 -> Add/1
  Saturation/1 -> Product/2, Add/2
  Add/1 -> Product1/2
  Product/1 -> Add1/2
  Product1/1 -> Add1/1
  In2/1 -> Product/1
  Add1/1 -> Out/1

== system base_1fm/Haptics/Hypotrochoid trajectory for AFFC/CrossFade5 ==
  In1 : Inport
  In2 : Inport  Port=2
  AmountIn2 : Inport  Port=3
  Add : Sum  Inputs=+-
  Add1 : Sum
  One : Constant
  Product : Product  RndMeth=Zero
  Product1 : Product  RndMeth=Zero
  Saturation : Saturate  UpperLimit=1  LowerLimit=0
  Out : Outport
  wires:
  In1/1 -> Product1/1
  AmountIn2/1 -> Saturation/1
  One/1 -> Add/1
  Saturation/1 -> Product/2, Add/2
  Add/1 -> Product1/2
  Product/1 -> Add1/2
  Product1/1 -> Add1/1
  In2/1 -> Product/1
  Add1/1 -> Out/1

== system base_1fm/Haptics/Hypotrochoid trajectory for AFFC/CrossFade6 ==
  In1 : Inport
  In2 : Inport  Port=2
  AmountIn2 : Inport  Port=3
  Add : Sum  Inputs=+-
  Add1 : Sum
  One : Constant
  Product : Product  RndMeth=Zero
  Product1 : Product  RndMeth=Zero
  Saturation : Saturate  UpperLimit=1  LowerLimit=0
  Out : Outport
  wires:
  In1/1 -> Product1/1
  AmountIn2/1 -> Saturation/1
  One/1 -> Add/1
  Saturation/1 -> Product/2, Add/2
  Add/1 -> Product1/2
  Product/1 -> Add1/2
  Product1/1 -> Add1/1
  In2/1 -> Product/1
  Add1/1 -> Out/1

== system base_1fm/Haptics/Hypotrochoid trajectory for AFFC/Cycloid ==
  note: Given a linear input 0<=in<=1, it gives a cycloid output 0<=out<=1.
      | If In is outside the 0..1 range, it is limited to 0 or 1.
  In : Inport
  Gain1 : Gain  Gain=2*pi
  Gain2 : Gain  Gain=1/(2*pi)
  Saturation : Saturate  UpperLimit=1  LowerLimit=0
  Subtract : Sum  Inputs=+-
  Trigonometric Function : Trigonometry
  Out : Outport
  wires:
  Gain1/1 -> Trigonometric Function/1
  Subtract/1 -> Out/1
  In/1 -> Saturation/1
  Saturation/1 -> Gain1/1, Subtract/1
  Trigonometric Function/1 -> Gain2/1
  Gain2/1 -> Subtract/2

== system base_1fm/Haptics/Hypotrochoid trajectory for AFFC/Cycloid1 ==
  note: Given a linear input 0<=in<=1, it gives a cycloid output 0<=out<=1.
      | If In is outside the 0..1 range, it is limited to 0 or 1.
  In : Inport
  Gain1 : Gain  Gain=2*pi
  Gain2 : Gain  Gain=1/(2*pi)
  Saturation : Saturate  UpperLimit=1  LowerLimit=0
  Subtract : Sum  Inputs=+-
  Trigonometric Function : Trigonometry
  Out : Outport
  wires:
  Gain1/1 -> Trigonometric Function/1
  Subtract/1 -> Out/1
  In/1 -> Saturation/1
  Saturation/1 -> Gain1/1, Subtract/1
  Trigonometric Function/1 -> Gain2/1
  Gain2/1 -> Subtract/2

== system base_1fm/Robot1/Controller/PD + Nonlinear ID ==
  q_ref : Inport
  qdot_ref : Inport  Port=2
  qddot_ref : Inport  Port=3
  RobotBus : Inport  Port=4
  systemState : Inport  Port=5
  AFFC : Subsystem
  Bus Creator : BusCreator  Inputs=4
  Bus Selector : BusSelector  OutputSignals=qJointSpace.q,qJointSpace.qdot
  Compare To Constant : simulink/Logic and Bit Operations/Compare To Constant  relop===  const=4  OutDataTypeStr=boolean
  DesiredTorque_PID : Display
  Gain : Gain
  Kd : Gain  Gain=0.1
  Kp : Gain  Gain=0.5
  Sum : Sum  Inputs=|+-
  Sum1 : Sum  Inputs=++|
  Sum2 : Sum  Inputs=|+-
  Sum3 : Sum  Inputs=|++
  p : Display
  JointTorqueDes_Nm : Outport
  ToLogger : Outport  Port=2
  wires:
  Bus Selector/2 -> Sum2/2  "<qdot>"
  Bus Selector/1 -> Sum/2  "<q>"
  q_ref/1 -> AFFC/1(q_ref), Sum/1
  Sum/1 -> Bus Creator/3, Kp/1  "e_p"
  Sum3/1 -> AFFC/4(e), Sum1/2
  Kd/1 -> Sum3/2
  Kp/1 -> Sum3/1
  qdot_ref/1 -> AFFC/2(qdot_ref), Sum2/1
  Sum2/1 -> Bus Creator/4, Kd/1  "e_d"
  Gain/1 -> Sum1/1
  Sum1/1 -> JointTorqueDes_Nm/1, DesiredTorque_PID/1
  RobotBus/1 -> Bus Selector/1
  qddot_ref/1 -> AFFC/3(qddot_ref)
  AFFC/1(p) -> Bus Creator/1, p/1  "p"
  AFFC/2(tau_affc) -> Bus Creator/2, Gain/1  "tau_affc"
  systemState/1 -> Compare To Constant/1
  Compare To Constant/1 -> AFFC/Enable
  Bus Creator/1 -> ToLogger/1  "ToLoggerPD"

== system base_1fm/Robot1/Controller/default ==
  Action Port : ActionPort  InitializeStates=reset
  Constant3 : Constant  Value=[0;0]
  JointTorqueDes_Nm : Outport  InitialOutput=[0;0]
  wires:
  Constant3/1 -> JointTorqueDes_Nm/1

== system base_1fm/Robot1/Controller/homing - active ==
  note: These blocks hold the first sample of the input
      | when the block is enabled (through the action port)
  HomePosition : Inport
  RobotBus : Inport  Port=2
  Action Port : ActionPort  InitializeStates=reset
  Bus Selector : BusSelector  OutputSignals=xOpSpace.x
  Constant1 : Constant
  Constant2 : Constant  Value=100*2*pi
  Constant4 : Constant  Value=[0;0]
  Counter Free-Running : simulink/Sources/Counter Free-Running  NumBits=32  tsamp=-1
  CrossFade : VariousBlocksLibrary/Various/CrossFade
  Cycloid : VariousBlocksLibrary/Various/Cycloid
  Discrete Derivative : simulink/Discrete/Discrete Derivative  gainval=1.0  ICPrevScaledInput=0.0  OutMin=[]  OutMax=[]  OutDataType=fixdt(1, 16)  OutScaling=2^-10  DoSatur=off
  Filter1 : MATLAB Function  AncestorBlock=WE1_library/FromActuator/ToJointAngle_rad/FilterFourthOrder/Filter1  TreatAsAtomicUnit=on  mask{sampleTime=sampleTime}
      mask prompts: sampleTime "Sample Time"
  Manual Switch : ManualSwitch  CurrentSetting=0
  Memory1 : Memory
  Rate Limiter : RateLimiter  RisingSlewLimit=0.2  FallingSlewLimit=-0.2  SampleTimeMode=inherited
  Switch : Switch  Threshold=1
  q_ref : Outport  InitialOutput=[0;0]
  qdot_ref : Outport  Port=2  InitialOutput=[0;0]
  qddot_ref : Outport  Port=3  InitialOutput=[0;0]
  wires:
  Constant4/1 -> qddot_ref/1
  CrossFade/1 -> Discrete Derivative/1, q_ref/1
  Manual Switch/1 -> CrossFade/1
  Memory1/1 -> Switch/1
  Counter Free-Running/1 -> Switch/2
  Switch/1 -> Manual Switch/1, Memory1/1
  Constant1/1 -> Rate Limiter/1
  Rate Limiter/1 -> Cycloid/1
  Cycloid/1 -> CrossFade/3
  HomePosition/1 -> CrossFade/2
  RobotBus/1 -> Bus Selector/1
  Bus Selector/1 -> Switch/3, Manual Switch/2  "<x>"
  Discrete Derivative/1 -> Filter1/1(x)
  Filter1/1(y) -> qdot_ref/1
  Constant2/1 -> Filter1/2(OmegaFilter)

== system base_1fm/Robot1/Controller/homing - done ==
  Action Port : ActionPort
  Constant : Constant  Value=[0;0]
  JointTorqueDes_Nm : Outport
  wires:
  Constant/1 -> JointTorqueDes_Nm/1

== system base_1fm/Robot1/Controller/idle (no torque) ==
  Action Port : ActionPort  InitializeStates=reset
  Constant3 : Constant  Value=[0;0]
  JointTorqueDes_Nm : Outport
  wires:
  Constant3/1 -> JointTorqueDes_Nm/1

== system base_1fm/Robot1/Controller/run ==
  q_ref_in : Inport
  qdot_ref_in : Inport  Port=2
  qddot_ref_in : Inport  Port=3
  Action Port : ActionPort  InitializeStates=reset
  q_ref : Outport
  qdot_ref : Outport  Port=2
  qddot_ref : Outport  Port=3
  wires:
  q_ref_in/1 -> q_ref/1
  qddot_ref_in/1 -> qddot_ref/1
  qdot_ref_in/1 -> qdot_ref/1

== system base_1fm/Robot1/Controller/velocity to zero ==
  note: Bring velocity down within 0.5 seconds
  note: These blocks hold the first sample of the input
      | when the block is enabled (through the action port)
  RobotBus : Inport
  Action Port : ActionPort  InitializeStates=reset  ActionType=case
  Add : Sum
  Bus Selector : BusSelector  OutputSignals=qJointSpace.q,qJointSpace.qdot
  Constant : Constant  Value=[0;0]
  Constant1 : Constant
  Constant2 : Constant  Value=[0;0]
  Counter Free-Running : simulink/Sources/Counter Free-Running  NumBits=32  tsamp=-1
  CrossFade : VariousBlocksLibrary/Various/CrossFade
  Cycloid : VariousBlocksLibrary/Various/Cycloid
  Discrete-Time Integrator : DiscreteIntegrator  InitialConditionSetting=State (most efficient)  SampleTime=-1  ICPrevOutput=DiscIntNeverNeededParam  ICPrevScaledInput=DiscIntNeverNeededParam
  Memory1 : Memory
  Rate Limiter : RateLimiter  RisingSlewLimit=2  FallingSlewLimit=-2  SampleTimeMode=inherited
  Switch : Switch  Threshold=1
  q_ref : Outport
  qdot_ref : Outport  Port=2
  qddot_ref : Outport  Port=3
  wires:
  RobotBus/1 -> Bus Selector/1
  Constant/1 -> qddot_ref/1
  Constant1/1 -> Rate Limiter/1
  Rate Limiter/1 -> Cycloid/1
  Cycloid/1 -> CrossFade/3
  CrossFade/1 -> Discrete-Time Integrator/1, qdot_ref/1
  Constant2/1 -> CrossFade/2
  Bus Selector/2 -> CrossFade/1  "<qdot>"
  Add/1 -> q_ref/1
  Discrete-Time Integrator/1 -> Add/2
  Memory1/1 -> Switch/1
  Counter Free-Running/1 -> Switch/2
  Switch/1 -> Add/1, Memory1/1
  Bus Selector/1 -> Switch/3  "<q>"

== system base_1fm/Robot1/DataFromEtherCAT/Calculate Arrange Joint and Op Space ==
  note: Here all angles of the parallel mechanism are calculated
      | based on the endpoint position, though this may still lead to incorrect
      | estimations of the internal angles (e.g. it is possible that on of the elbows
      | has gone through a singular position already). So perhaps I should also include
      | a different way of calculating the internal angles
  BusActuators : Inport
  Bus Creator1 : BusCreator  Inputs=3
  Bus Creator2 : BusCreator  Inputs=3
  Bus Selector : BusSelector  OutputSignals=BusActuator1.JointPosition_rad,BusActuator2.JointPosition_rad  OutputAsBus=on
  Bus Selector1 : BusSelector  OutputSignals=BusActuator1.JointVelocity_rads,BusActuator2.JointVelocity_rads  OutputAsBus=on
  Bus Selector2 : BusSelector  OutputSignals=BusActuator1.JointPosition_rad,BusActuator2.JointPosition_rad,BusActuator1.JointVelocity_rads,BusActuator2.JointVelocity_rads
  Ground : Ground
  IK all joints : MATLAB Function  TreatAsAtomicUnit=on
  Mux : Mux  Inputs=2
  Mux1 : Mux  Inputs=2
  Terminator1 : Terminator
  Terminator2 : Terminator
  forward kinematics : Subsystem
  xOpSpace : Outport
  qJointSpace : Outport  Port=2
  wires:
  IK all joints/1(q_all) -> Bus Creator2/3  "qall"
  Mux1/1 -> Bus Creator2/2  "qdot"
  Bus Selector2/4 -> Mux1/2  "<JointVelocity_rads>"
  Bus Selector2/3 -> Mux1/1  "<JointVelocity_rads>"
  Bus Selector2/2 -> Mux/2  "<JointPosition_rad>"
  Bus Selector2/1 -> Mux/1  "<JointPosition_rad>"
  Mux/1 -> Bus Creator2/1  "q"
  BusActuators/1 -> Bus Selector/1, Bus Selector2/1, Bus Selector1/1
  Bus Creator2/1 -> qJointSpace/1  "JointSpace"
  Ground/1 -> forward kinematics/3(JointAcceleration_rads2)
  Bus Selector1/1 -> forward kinematics/2(JointVelocity_rads)
  forward kinematics/4(J) -> Bus Creator1/3  "jacobian"
  Bus Creator1/1 -> xOpSpace/1  "OpSpace"
  forward kinematics/1(x) -> Bus Creator1/1, IK all joints/1(x)  "x"
  Bus Selector/1 -> forward kinematics/1(JointPosition_rad)
  forward kinematics/2(xdot) -> Bus Creator1/2  "xdot"
  forward kinematics/3(xddot) -> Terminator1/1
  forward kinematics/5(Jdot) -> Terminator2/1

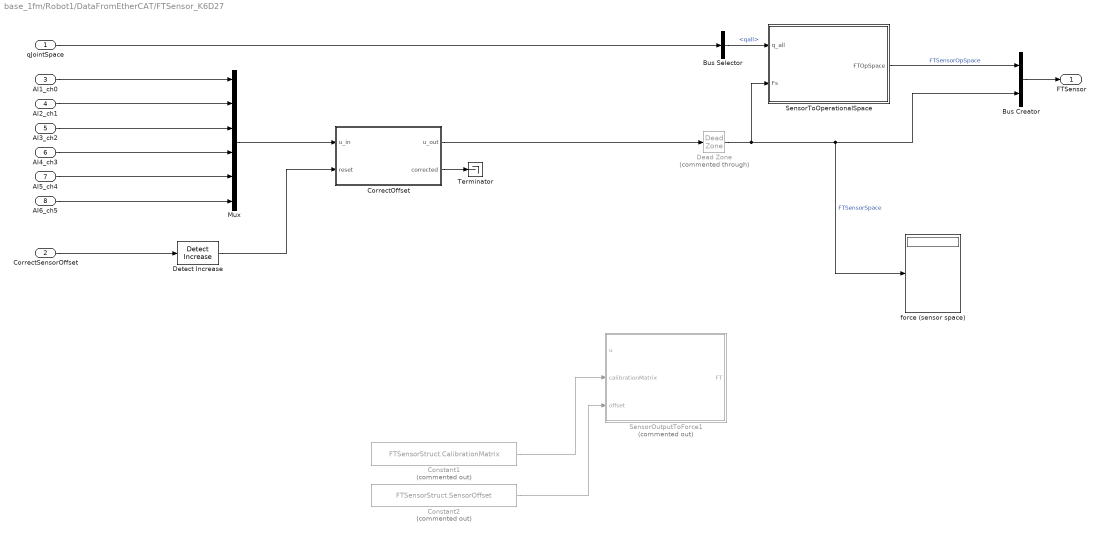
== system base_1fm/Robot1/DataFromEtherCAT/FTSensor_K6D27 ==
  qJointSpace : Inport
  CorrectSensorOffset : Inport  Port=2
  AI1_ch0 : Inport  Port=3  OutDataTypeStr=int16
  AI2_ch1 : Inport  Port=4  OutDataTypeStr=int16
  AI3_ch2 : Inport  Port=5  OutDataTypeStr=int16
  AI4_ch3 : Inport  Port=6  OutDataTypeStr=int16
  AI5_ch4 : Inport  Port=7  OutDataTypeStr=int16
  AI6_ch5 : Inport  Port=8  OutDataTypeStr=int16
  Bus Creator : BusCreator  Inputs=2
  Bus Selector : BusSelector  OutputSignals=qall
  Constant1 : Constant  Commented=on  Value=FTSensorStruct.CalibrationMatrix
  Constant2 : Constant  Commented=on  Value=FTSensorStruct.SensorOffset
  CorrectOffset : MATLAB Function  TreatAsAtomicUnit=on
  Dead Zone : DeadZone  Commented=through  LowerValue=-0.05  UpperValue=0.05  SaturateOnIntegerOverflow=on
  Detect Increase : simulink/Logic and Bit Operations/Detect Increase  vinit=0.0  InputProcessing=Inherited  OutDataTypeStr=boolean
  Mux : Mux  Inputs=6
  SensorOutputToForce1 : MATLAB Function  Commented=on  TreatAsAtomicUnit=on
  SensorToOperationalSpace : MATLAB Function  TreatAsAtomicUnit=on
  Terminator : Terminator
  force (sensor space) : Display
  FTSensor : Outport
  wires:
  SensorToOperationalSpace/1(FTOpSpace) -> Bus Creator/1  "FTSensorOpSpace"
  Bus Creator/1 -> FTSensor/1
  Dead Zone/1 -> SensorToOperationalSpace/2(Fs), force (sensor space)/1, Bus Creator/2  "FTSensorSpace"
  CorrectOffset/2(corrected) -> Terminator/1
  AI3_ch2/1 -> Mux/3
  AI4_ch3/1 -> Mux/4
  AI5_ch4/1 -> Mux/5
  AI6_ch5/1 -> Mux/6
  Bus Selector/1 -> SensorToOperationalSpace/1(q_all)  "<qall>"
  CorrectOffset/1(u_out) -> Dead Zone/1
  Detect Increase/1 -> CorrectOffset/2(reset)
  CorrectSensorOffset/1 -> Detect Increase/1
  Mux/1 -> CorrectOffset/1(u_in)
  AI1_ch0/1 -> Mux/1
  AI2_ch1/1 -> Mux/2
  qJointSpace/1 -> Bus Selector/1
  Constant2/1 -> SensorOutputToForce1/3(offset)
  Constant1/1 -> SensorOutputToForce1/2(calibrationMatrix)

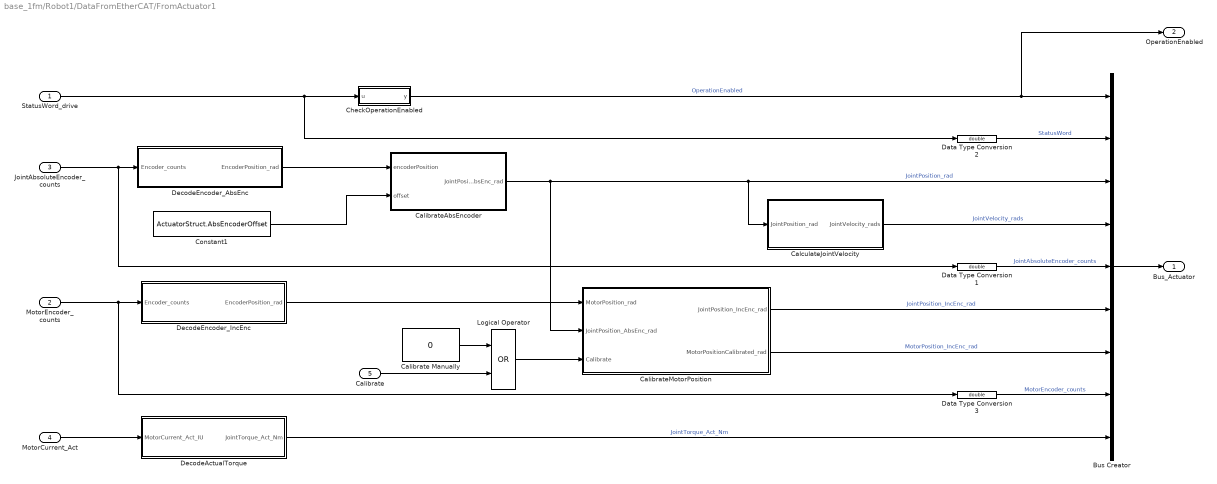
== system base_1fm/Robot1/DataFromEtherCAT/FromActuator1 ==
  StatusWord_drive : Inport
  MotorEncoder_counts : Inport  Port=2
  JointAbsoluteEncoder_counts : Inport  Port=3
  MotorCurrent_Act : Inport  Port=4
  Calibrate : Inport  Port=5
  Bus Creator : BusCreator  Inputs=9
  CalculateJointVelocity : Subsystem
  Calibrate Manually : Constant  Value=0
      settings: OpenFcn=set_param(gcb,'Value','1');tname = ['toggletimer_' gcb];delete(timerfind('name',tname));t = timer('timerfcn', ['set_param(''',gcb,''',''Value'',''0'')'],'executionmode','singleshot','startdelay',1,'name',tname);start(t);
      mask Display: fprintf('PushToTrigger\n%s',get_param(gcb,'value'))
  CalibrateAbsEncoder : MATLAB Function  TreatAsAtomicUnit=on
  "CalibrateMotorPosition    " : MATLAB Function  TreatAsAtomicUnit=on  mask{gearboxRatio=ActuatorStruct.transmissionRatio}
      mask prompts: gearboxRatio "Transmission ratio (e.g. -8) [-]"
  CheckOperationEnabled : MATLAB Function  TreatAsAtomicUnit=on
  Constant1 : Constant  Value=ActuatorStruct.AbsEncoderOffset
  Data Type Conversion1 : DataTypeConversion  OutDataTypeStr=double
  Data Type Conversion2 : DataTypeConversion  OutDataTypeStr=double
  Data Type Conversion3 : DataTypeConversion  OutDataTypeStr=double
  DecodeActualTorque : MATLAB Function  TreatAsAtomicUnit=on  mask(DecodeActualTorque){transmissionRatio=ActuatorStruct.transmissionRatio, motorTorqueConstant=ActuatorStruct.motorTorqueConstant, drivePeakCurrent=ActuatorStruct.drivePeakCurrent}
      mask prompts: transmissionRatio "Transmission ratio (e.g. -8) [-]"; motorTorqueConstant "Motor torque constant [Nm/A]"; drivePeakCurrent "Motor drive peak current Ipeak [A]"
      mask help:
      | Decode Actual Torque value returned from the actuator (motor drive and motor) to torque on the joint (after transmission).
      |
      | Note: due to the way the transmission is set up and the positive motor axis (clockwise is positive as seen from the motor front), there is no need to account for sign change in motor torque or encoder position.
  DecodeEncoder_AbsEnc : MATLAB Function  TreatAsAtomicUnit=on  mask(DecodeEncoder){EncoderCounts_rev=ActuatorStruct.JointAbsoluteEncoderCounts_rev}
      mask prompts: EncoderCounts_rev "Motor encoder increments per revolution (e.g., 8192)"
      mask help: Decode the encoder counts to encoder position in radians
  DecodeEncoder_IncEnc : MATLAB Function  TreatAsAtomicUnit=on  mask(DecodeEncoder){EncoderCounts_rev=ActuatorStruct.MotorEncoderCounts_rev}
      mask prompts: EncoderCounts_rev "Motor encoder increments per revolution (e.g., 8192)"
      mask help: Decode the encoder counts to encoder position in radians
  Logical Operator : Logic  Operator=OR  AllPortsSameDT=off  OutDataTypeStr=boolean
  Bus_Actuator : Outport
  OperationEnabled : Outport  Port=2
  wires:
  Calibrate Manually/1 -> Logical Operator/1
  Constant1/1 -> CalibrateAbsEncoder/2(offset)
  Logical Operator/1 -> "CalibrateMotorPosition    "/3(Calibrate)
  Bus Creator/1 -> Bus_Actuator/1
  Data Type Conversion3/1 -> Bus Creator/8  "MotorEncoder_counts"
  MotorEncoder_counts/1 -> Data Type Conversion3/1, DecodeEncoder_IncEnc/1(Encoder_counts)
  CalibrateAbsEncoder/1(JointPosition_AbsEnc_rad) -> Bus Creator/3, CalculateJointVelocity/1(JointPosition_rad), "CalibrateMotorPosition    "/2(JointPosition_AbsEnc_rad)  "JointPosition_rad"
  Data Type Conversion2/1 -> Bus Creator/2  "StatusWord"
  Data Type Conversion1/1 -> Bus Creator/5  "JointAbsoluteEncoder_counts"
  "CalibrateMotorPosition    "/1(JointPosition_IncEnc_rad) -> Bus Creator/6  "JointPosition_IncEnc_rad"
  JointAbsoluteEncoder_counts/1 -> DecodeEncoder_AbsEnc/1(Encoder_counts), Data Type Conversion1/1
  CheckOperationEnabled/1(y) -> Bus Creator/1, OperationEnabled/1  "OperationEnabled"
  MotorCurrent_Act/1 -> DecodeActualTorque/1(MotorCurrent_Act_IU)
  DecodeEncoder_IncEnc/1(EncoderPosition_rad) -> "CalibrateMotorPosition    "/1(MotorPosition_rad)
  StatusWord_drive/1 -> CheckOperationEnabled/1(u), Data Type Conversion2/1
  DecodeActualTorque/1(JointTorque_Act_Nm) -> Bus Creator/9  "JointTorque_Act_Nm"
  "CalibrateMotorPosition    "/2(MotorPositionCalibrated_rad) -> Bus Creator/7  "MotorPosition_IncEnc_rad"
  DecodeEncoder_AbsEnc/1(EncoderPosition_rad) -> CalibrateAbsEncoder/1(encoderPosition)
  CalculateJointVelocity/1(JointVelocity_rads) -> Bus Creator/4  "JointVelocity_rads"
  Calibrate/1 -> Logical Operator/2

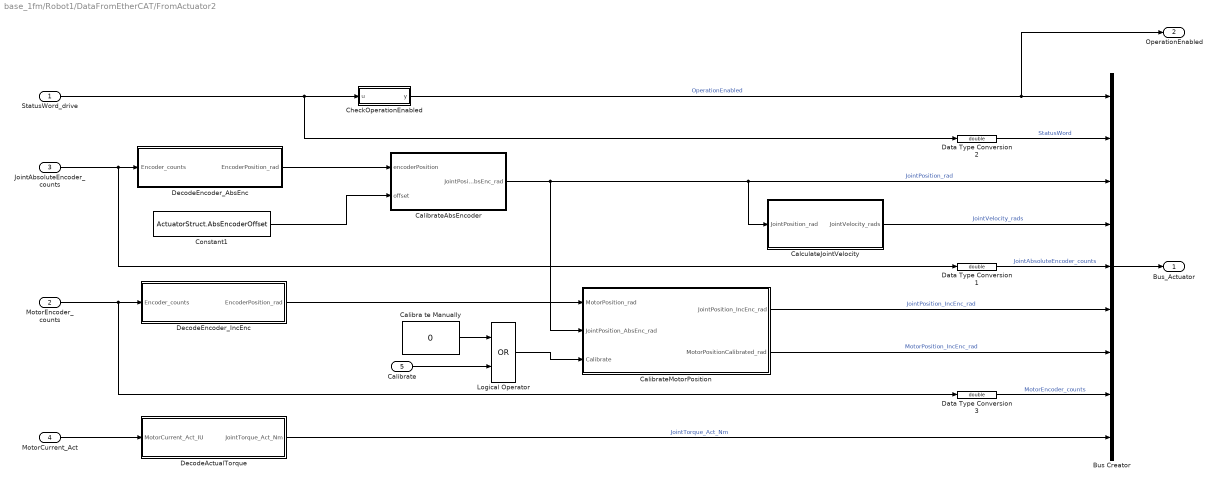
== system base_1fm/Robot1/DataFromEtherCAT/FromActuator2 ==
  StatusWord_drive : Inport
  MotorEncoder_counts : Inport  Port=2
  JointAbsoluteEncoder_counts : Inport  Port=3
  MotorCurrent_Act : Inport  Port=4
  Calibrate : Inport  Port=5
  Bus Creator : BusCreator  Inputs=9
  CalculateJointVelocity : Subsystem
  Calibra te Manually : Constant  Value=0
      settings: OpenFcn=set_param(gcb,'Value','1');tname = ['toggletimer_' gcb];delete(timerfind('name',tname));t = timer('timerfcn', ['set_param(''',gcb,''',''Value'',''0'')'],'executionmode','singleshot','startdelay',1,'name',tname);start(t);
      mask Display: fprintf('PushToTrigger\n%s',get_param(gcb,'value'))
  CalibrateAbsEncoder : MATLAB Function  TreatAsAtomicUnit=on
  "CalibrateMotorPosition    " : MATLAB Function  TreatAsAtomicUnit=on  mask{gearboxRatio=ActuatorStruct.transmissionRatio}
      mask prompts: gearboxRatio "Transmission ratio (e.g. -8) [-]"
  CheckOperationEnabled : MATLAB Function  TreatAsAtomicUnit=on
  Constant1 : Constant  Value=ActuatorStruct.AbsEncoderOffset
  Data Type Conversion1 : DataTypeConversion  OutDataTypeStr=double
  Data Type Conversion2 : DataTypeConversion  OutDataTypeStr=double
  Data Type Conversion3 : DataTypeConversion  OutDataTypeStr=double
  DecodeActualTorque : MATLAB Function  TreatAsAtomicUnit=on  mask(DecodeActualTorque){transmissionRatio=ActuatorStruct.transmissionRatio, motorTorqueConstant=ActuatorStruct.motorTorqueConstant, drivePeakCurrent=ActuatorStruct.drivePeakCurrent}
      mask prompts: transmissionRatio "Transmission ratio (e.g. -8) [-]"; motorTorqueConstant "Motor torque constant [Nm/A]"; drivePeakCurrent "Motor drive peak current Ipeak [A]"
      mask help:
      | Decode Actual Torque value returned from the actuator (motor drive and motor) to torque on the joint (after transmission).
      |
      | Note: due to the way the transmission is set up and the positive motor axis (clockwise is positive as seen from the motor front), there is no need to account for sign change in motor torque or encoder position.
  DecodeEncoder_AbsEnc : MATLAB Function  TreatAsAtomicUnit=on  mask(DecodeEncoder){EncoderCounts_rev=ActuatorStruct.JointAbsoluteEncoderCounts_rev}
      mask prompts: EncoderCounts_rev "Motor encoder increments per revolution (e.g., 8192)"
      mask help: Decode the encoder counts to encoder position in radians
  DecodeEncoder_IncEnc : MATLAB Function  TreatAsAtomicUnit=on  mask(DecodeEncoder){EncoderCounts_rev=ActuatorStruct.MotorEncoderCounts_rev}
      mask prompts: EncoderCounts_rev "Motor encoder increments per revolution (e.g., 8192)"
      mask help: Decode the encoder counts to encoder position in radians
  Logical Operator : Logic  Operator=OR  AllPortsSameDT=off  OutDataTypeStr=boolean
  Bus_Actuator : Outport
  OperationEnabled : Outport  Port=2
  wires:
  Calibra te Manually/1 -> Logical Operator/1
  Constant1/1 -> CalibrateAbsEncoder/2(offset)
  Logical Operator/1 -> "CalibrateMotorPosition    "/3(Calibrate)
  Bus Creator/1 -> Bus_Actuator/1
  Data Type Conversion3/1 -> Bus Creator/8  "MotorEncoder_counts"
  MotorEncoder_counts/1 -> Data Type Conversion3/1, DecodeEncoder_IncEnc/1(Encoder_counts)
  CalibrateAbsEncoder/1(JointPosition_AbsEnc_rad) -> Bus Creator/3, CalculateJointVelocity/1(JointPosition_rad), "CalibrateMotorPosition    "/2(JointPosition_AbsEnc_rad)  "JointPosition_rad"
  Data Type Conversion2/1 -> Bus Creator/2  "StatusWord"
  Data Type Conversion1/1 -> Bus Creator/5  "JointAbsoluteEncoder_counts"
  "CalibrateMotorPosition    "/1(JointPosition_IncEnc_rad) -> Bus Creator/6  "JointPosition_IncEnc_rad"
  JointAbsoluteEncoder_counts/1 -> DecodeEncoder_AbsEnc/1(Encoder_counts), Data Type Conversion1/1
  CheckOperationEnabled/1(y) -> Bus Creator/1, OperationEnabled/1  "OperationEnabled"
  MotorCurrent_Act/1 -> DecodeActualTorque/1(MotorCurrent_Act_IU)
  DecodeEncoder_IncEnc/1(EncoderPosition_rad) -> "CalibrateMotorPosition    "/1(MotorPosition_rad)
  StatusWord_drive/1 -> CheckOperationEnabled/1(u), Data Type Conversion2/1
  DecodeActualTorque/1(JointTorque_Act_Nm) -> Bus Creator/9  "JointTorque_Act_Nm"
  "CalibrateMotorPosition    "/2(MotorPositionCalibrated_rad) -> Bus Creator/7  "MotorPosition_IncEnc_rad"
  DecodeEncoder_AbsEnc/1(EncoderPosition_rad) -> CalibrateAbsEncoder/1(encoderPosition)
  CalculateJointVelocity/1(JointVelocity_rads) -> Bus Creator/4  "JointVelocity_rads"
  Calibrate/1 -> Logical Operator/2

== system base_1fm/Robot1/DataToEtherCAT/FTSensorError ==
  RobotBus : Inport
  AvoidAlgebraicLoop : Memory
  Bus Selector1 : BusSelector  OutputSignals=FTSensor.FTSensorSpace
  Constant : Constant  Value=RobotStruct.MaxAllowableForcesTorqueSensor
  CreateSingleErrorValue : FMLibrary_v2/DataToEtherCAT_FM/WorkspacePositionGuard/CreateSingleErrorValue
  Detect Change : simulink/Logic and Bit Operations/Detect Change  vinit=0  InputProcessing=Inherited  OutDataTypeStr=boolean
  FTSensorLastError : Display
  LatchRising : UsefulBlocksLibrary/LatchRising  ic=0
  MATLAB Function : MATLAB Function  TreatAsAtomicUnit=on
  ShowFTSensorErrorLatched : Display
  FTSensorError : Outport
  FTSensorErrorLatched : Outport  Port=2
  wires:
  Constant/1 -> MATLAB Function/2(MaxForcesTorques)
  MATLAB Function/1(e) -> FTSensorLastError/1, CreateSingleErrorValue/1
  Bus Selector1/1 -> MATLAB Function/1(ForcesTorques)  "<FTSensorSpace>"
  RobotBus/1 -> Bus Selector1/1
  CreateSingleErrorValue/1 -> AvoidAlgebraicLoop/1
  LatchRising/1 -> ShowFTSensorErrorLatched/1, FTSensorErrorLatched/1
  AvoidAlgebraicLoop/1 -> LatchRising/1, Detect Change/1, FTSensorError/1
  Detect Change/1 -> LatchRising/Trigger
